simulink model "arduino_CAN_packandunpack_example"  (R2017b)
settings: Solver=FixedStepDiscrete  StartTime=0.0  StopTime=10.0  FixedStep=0.1  RelTol=1e-3  EnableMultiTasking=on
libraries: arduino_CAN_library x3, arduinolib x2, canmsglib x1, simulink x1
settings Model: ExtModeTrigDuration=2  Creator=ll2  LastModifiedBy=ll2
settings DataIOCC: SaveFormat=StructureWithTime
settings OptimizationCC: BlockReduction=off  PassReuseOutputArgsAs=Individual arguments  LifeSpan=inf  MaxStackSize=64
settings DebuggingCC: ParameterTunabilityLossMsg=error  SFExecutionAtInitializationDiag=none
settings HardwareCC: ProdBitPerInt=16  ProdBitPerPointer=8  ProdBitPerSizeT=16  ProdBitPerPtrDiffT=16  ProdLargestAtomicFloat=None  ProdWordSize=8  ProdHWDeviceType=Atmel->AVR
settings SFSimCC: MATLABDynamicMemAlloc=off
settings RTWCC: SystemTargetFile=ert.tlc  HardwareBoard=Arduino Uno  TLCOptions=-aInlineSetEventsForThisBaseRateFcn=TLC_FALSE -aSuppressMultiTaskScheduler=TLC_FALSE -aRateBasedStepFcn=1  TemplateMakefile=ert_default_tmf  GenerateReport=on  RTWVerbose=off  CustomInclude="\"..\\..\\externals\\CAN-Bus_Shield\\Libraries\\Canbus\""  CustomSource="\"..\\..\\externals\\CAN-Bus_Shield\\Libraries\\Canbus\\mcp2515.c\""  Toolchain=Arduino AVR  BuildConfiguration=Faster Runs  IncludeHyperlinkInReport=on  LaunchReport=on  GenerateTraceInfo=on  GenerateTraceReport=on  GenerateTraceReportSl=on  GenerateTraceReportSf=on  GenerateTraceReportEml=on
settings CodeAppCC: ForceParamTrailComments=on  IgnoreCustomStorageClasses=off  OperatorAnnotations=on  SimulinkDataObjDesc=on  SFDataObjDesc=on  InsertBlockDesc=on  StateflowObjectComments=on
settings ERTTargetCC: SupportContinuousTime=on  SupportVariableSizeSignals=on

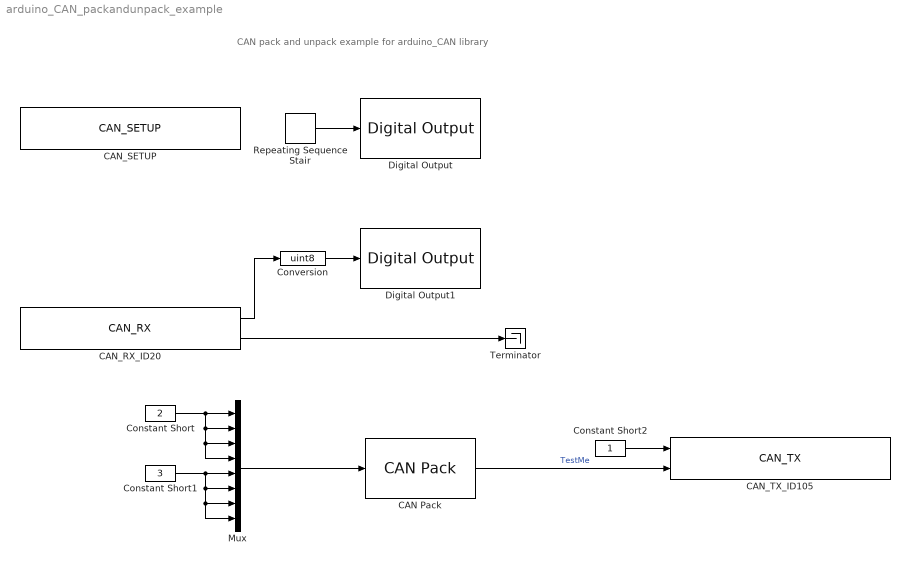
== system arduino_CAN_packandunpack_example ==
  note: CAN pack and unpack example for arduino_CAN library
  CAN Pack : canmsglib/CAN Pack  MsgList=(none)  MsgName=CANMsg_ID105  MsgIDType=Standard (11-bit identifier)  MsgIdentifier=0  MsgLength=8  NSignals=0  StartBits=0  SignalSizes=0  ByteOrders=0  DataTypes=0  MultiplexTypes=0  MultiplexValues=0  Factors=0  Offsets=0  Minimums=0  Maximums=0  Remote=off  ApplyMinMax=off  BusOutput=off
      settings: SourceProductName=Simulink Real-Time  SourceProductBaseCode=XP  DataFormat=raw data
  CAN_RX_ID20 : arduino_CAN_library/CAN_RX  CANM_ID=20
  CAN_SETUP : arduino_CAN_library/CAN_SETUP  CANIDX=250
  CAN_TX_ID105 : arduino_CAN_library/CAN_TX  CANM_ID=105  CANM_DTYPE=CAN_MESSAGE
  Constant Short : Constant  Value=2  OutDataTypeStr=uint8
  Constant Short1 : Constant  Value=3  OutDataTypeStr=uint8
  Constant Short2 : Constant  OutDataTypeStr=uint8
  Conversion : DataTypeConversion  OutDataTypeStr=uint8
  Digital Output : arduinolib/Digital Output  pinNumber=7  blockPlatform=arduino
  Digital Output1 : arduinolib/Digital Output  pinNumber=8  blockPlatform=arduino
  Mux : Mux  Inputs=8
  Repeating Sequence Stair : simulink/Sources/Repeating Sequence Stair  OutValues=[1 1 0 1 0 0 1 1 1 1 1 1 1].'  tsamp=0.1  OutMin=[]  OutMax=[]  OutDataTypeStr=uint8  OutputDataTypeScalingMode=uint8  OutDataType=double  ConRadixGroup=Best Precision: Vector-wise  OutScaling=2^-12
  Terminator : Terminator
  wires:
  Constant Short/1 -> Mux/1, Mux/2, Mux/3, Mux/4
  Conversion/1 -> Digital Output1/1
  Constant Short2/1 -> CAN_TX_ID105/1
  Repeating Sequence Stair/1 -> Digital Output/1
  CAN_RX_ID20/1 -> Conversion/1
  Constant Short1/1 -> Mux/5, Mux/6, Mux/7, Mux/8
  CAN_RX_ID20/2 -> Terminator/1
  Mux/1 -> CAN Pack/1
  CAN Pack/1 -> CAN_TX_ID105/2  "TestMe"
